simulink model "Dfig"  (R2014a)
settings: Solver=ode45  StartTime=0.0  StopTime=3.5  RelTol=1e-3
values from neighbouring files (symbols this model uses):
  Cbus = 80e-3    (= 0.08)    [Parameter_2M_DFIG.m]    (also in Parameter_2M_DFIG_GSC.m; ini2.m; init.m)
  D = 1e-3    (= 0.001)    [Parameter_2M_DFIG.m]    (also in Parameter_2M_DFIG_GSC.m = 0.1; ini.m; ini2.m; init.m)
  f = 50    [Parameter_2M_DFIG.m]    (also in Parameter_2M_DFIG_GSC.m = 60; ini.m; ini2.m; init.m)
  Fs = 1.28    [Parameter_2M_DFIG.m]    (also in Parameter_2M_DFIG_GSC.m = 1.8; ini.m = Vs*sqrt(2/3)/(2*pi*f); ini2.m = Vs*sqrt(2/3)/(2*pi*f); init.m = Vs*sqrt(2/3)/(2*pi*f))
  fsw = 4e3    (= 4000)    [Parameter_2M_DFIG.m]    (also in Parameter_2M_DFIG_GSC.m; ini.m; ini2.m; init.m)
  J = 127    [Parameter_2M_DFIG.m]    (also in Parameter_2M_DFIG_GSC.m = 90; ini.m; ini2.m; init.m)
  ki_id = (wni^2)*Lr*sigma    (= 491.599501999)    [Parameter_2M_DFIG.m]    (also in Parameter_2M_DFIG_GSC.m; ini.m; ini2.m; init.m)
  ki_idg = (wnig^2)*Lg    (= 68.6450725305)    [Parameter_2M_DFIG.m]    (also in Parameter_2M_DFIG_GSC.m; ini2.m = 56.8489213503; init.m = 56.8489213503)
  ki_iq = ki_id    (= 491.599501999)    [Parameter_2M_DFIG.m]    (also in Parameter_2M_DFIG_GSC.m; ini.m; ini2.m; init.m)
  ki_iqg = ki_idg    (= 68.6450725305)    [Parameter_2M_DFIG.m]    (also in Parameter_2M_DFIG_GSC.m; ini2.m = 56.8489213503; init.m = 56.8489213503)
  ki_n = ((wnn^2)*J)/p    (= 25400)    [Parameter_2M_DFIG.m]    (also in Parameter_2M_DFIG_GSC.m = 18000; ini.m; ini2.m; init.m)
  kp_id = (2*wni*sigma*Lr)-Rr    (= 0.5771)    [Parameter_2M_DFIG.m]    (also in Parameter_2M_DFIG_GSC.m; ini.m; ini2.m; init.m)
  kp_idg = (2*wnig*Lg)-Rg    (= 0.364153420404)    [Parameter_2M_DFIG.m]    (also in Parameter_2M_DFIG_GSC.m; ini2.m = 0.301572894745; init.m = 0.301572894745)
  kp_iq = kp_id    (= 0.5771)    [Parameter_2M_DFIG.m]    (also in Parameter_2M_DFIG_GSC.m; ini.m; ini2.m; init.m)
  kp_iqg = kp_idg    (= 0.364153420404)    [Parameter_2M_DFIG.m]    (also in Parameter_2M_DFIG_GSC.m; ini2.m = 0.301572894745; init.m = 0.301572894745)
  kp_n = (2*wnn*J)/p    (= 2540)    [Parameter_2M_DFIG.m]    (also in Parameter_2M_DFIG_GSC.m = 1800; ini.m; ini2.m; init.m)
  Kpg = 1/(1.5*Vs*sqrt(2/3))    [Parameter_2M_DFIG.m]    (also in Parameter_2M_DFIG_GSC.m; ini2.m; init.m)
  Kqg = -Kpg    [Parameter_2M_DFIG.m]    (also in Parameter_2M_DFIG_GSC.m; ini2.m; init.m)
  Lg = 483e-6    (= 0.000483)    [Parameter_2M_DFIG.m]    (also in Parameter_2M_DFIG_GSC.m; ini2.m = 0.0004; init.m = 0.0004)
  Lm = 2.5e-3    (= 0.0025)    [Parameter_2M_DFIG.m]    (also in Parameter_2M_DFIG_GSC.m; ini.m; ini2.m; init.m)
  Lr = Lm + Lsr    (= 0.002587)    [Parameter_2M_DFIG.m]    (also in Parameter_2M_DFIG_GSC.m; ini.m; ini2.m; init.m)
  Ls = Lm + Lsi    (= 0.002587)    [Parameter_2M_DFIG.m]    (also in Parameter_2M_DFIG_GSC.m; ini.m; ini2.m; init.m)
  Lsi = 87e-6    (= 8.7e-05)    [Parameter_2M_DFIG.m]    (also in Parameter_2M_DFIG_GSC.m; ini.m; ini2.m; init.m)
  N = 100    [Parameter_2M_DFIG.m]    (also in Parameter_2M_DFIG_GSC.m; ini2.m; init.m)
  p = 2    [Parameter_2M_DFIG.m]    (also in Parameter_2M_DFIG_GSC.m; ini.m; ini2.m; init.m)
  Ps = 2e6    (= 2000000)    [Parameter_2M_DFIG.m]    (also in Parameter_2M_DFIG_GSC.m; ini.m; ini2.m; init.m)
  Rg = 20e-6    (= 2e-05)    [Parameter_2M_DFIG.m]    (also in Parameter_2M_DFIG_GSC.m; ini2.m; init.m)
  Rr = 2.9e-3    (= 0.0029)    [Parameter_2M_DFIG.m]    (also in Parameter_2M_DFIG_GSC.m; ini.m; ini2.m; init.m)
  Rs = 2.6e-3    (= 0.0026)    [Parameter_2M_DFIG.m]    (also in Parameter_2M_DFIG_GSC.m; ini.m; ini2.m; init.m)
  sigma = 1- Lm^2/(Ls*Lr)    (= 0.0661284179513)    [Parameter_2M_DFIG.m]    (also in Parameter_2M_DFIG_GSC.m; ini.m; ini2.m; init.m)
  Tem = 12732    [Parameter_2M_DFIG.m]    (also in Parameter_2M_DFIG_GSC.m; ini.m; ini2.m; init.m)
  Ts = 1/fsw/f    (= 5e-06)    [Parameter_2M_DFIG.m]    (also in Parameter_2M_DFIG_GSC.m = 4.16666666667e-06; ini.m; ini2.m; init.m)
  Vbus = 1000    [Parameter_2M_DFIG.m]    (also in ini.m = Vr_stator*sqrt(2); ini2.m = 1150; init.m = 1150)
  Vs = 690    [Parameter_2M_DFIG.m]    (also in Parameter_2M_DFIG_GSC.m; ini.m; ini2.m; init.m)
undefined symbols (not defined in the file or in its folder): c1, c2, c3, c4, c5, c6, c7, c8, Ct, DiscIntNeverNeededParam, K1, K2
libraries: powerlib x18, powerlib_meascontrol x5, simulink x1
settings Model: CovSFcnEnable=on  Creator=admin  LastModifiedBy=admin
settings DebuggingCC: UnderspecifiedInitializationDetection=Classic  FrameProcessingCompatibilityMsg=error  StateNameClashWarn=warning
settings SimscapeCC: SimscapeNormalizeSystem=off
settings ConfigurationSet: Description=Simscape Multibody

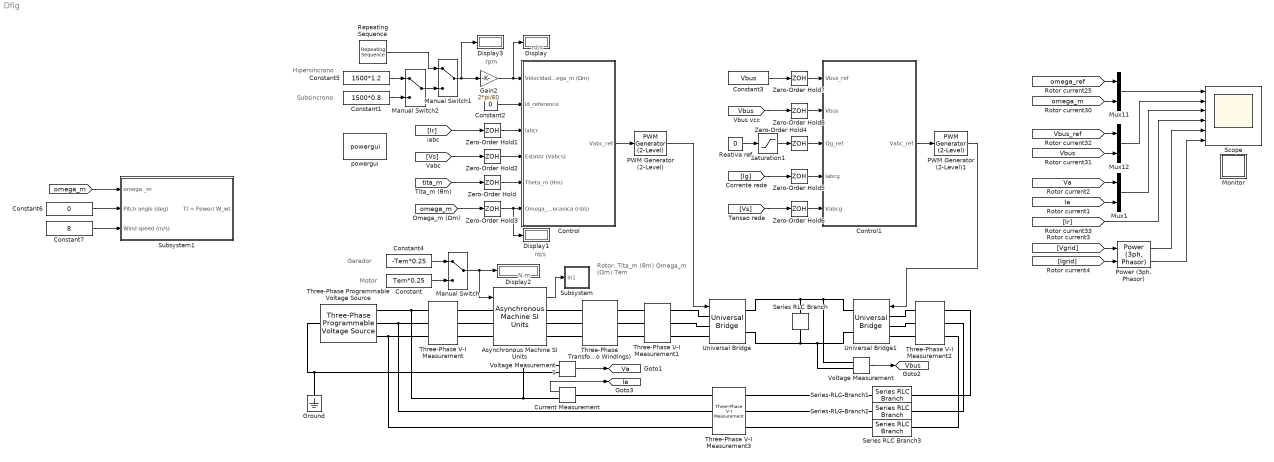
== system Dfig ==
  note: N.m
  note: Gerador
  note: Motor
  note: rd/s
  note: rpm
  note: Rotor:
      | Tita_m (θm)
      | Omega_m (Ωm)
      | Tem
  note: rd/s
  note: Hipersincrono
  note: Subsincrono
  Asynchronous Machine SI Units : powerlib/Machines/Asynchronous Machine SI Units  RotorType=Wound  PresetModel=No  MechanicalLoad=Torque Tm  ShowDetailedParameters=on  ReferenceFrame=Rotor  Units=SI  MeasurementBus=off  NominalParameters=[ Ps Vs f ]  Stator=[ Rs , Lsi]  Rotor=[ Rr , Lsi]  Cage1=[ 0.022 0.226/377]  Cage2=[ 0.022 0.226/377]  Lm=Lm  Mechanical=[ J D 2 ]  PolePairs=2  InitialConditions=[1 0 0 0 0 0 0 0]  SimulateSaturation=off  Saturation=[14.03593122, 27.81365428, 53.79336849, 72.68890987, 97.98006896, 148.6815601, 215.7428561, 302.9841135, 420.4778367 ; 230, 322, 414, 460, 506, 552, 598, 644, 690]  LoadFlowParameters=1492000  TsPowergui=0  TsBlock=-1  IterativeModel=Trapezoidal non iterative  IterativeDiscreteModel=Trapezoidal non iterative  Pmec=0
  Constant : Constant  Value=Tem*0.25
  Constant1 : Constant  Value=1500*0.8
  Constant2 : Constant  Value=0
  Constant3 : Constant  Value=Vbus
  Constant4 : Constant  Value=-Tem*0.25
  Constant5 : Constant  Value=1500*1.2
  Constant6 : Constant  Value=0
  Constant7 : Constant  Value=8
  Control : Subsystem
  Control1 : Subsystem
  Current Measurement : powerlib/Measurements/Current Measurement  PhasorSimulation=off  OutputType=Complex  PSBequivalent=0
  Display{,1..3} (4 alike) : Display
  Gain2 : Gain  Gain=2*pi/60
  Ground : powerlib/Elements/Ground  LConnTagsString=a
  Manual Switch : ManualSwitch
  Manual Switch1 : ManualSwitch
  Manual Switch2 : ManualSwitch
  Monitor : Subsystem
  Mux1 : Mux  Inputs=2
  Mux11 : Mux  Inputs=2
  Mux12 : Mux  Inputs=2
  PWM Generator (2-Level) : powerlib_meascontrol/Pulse & Signal Generators/PWM Generator (2-Level)  ModulatorType=Three-phase bridge (6 pulses)  ModulatorMode=Unsynchronized  Fc=fsw  Pc=0  nF=27  MinMax="[ -1  1 ]"  SamplingTechnique=Natural  ModulatingSignals=off  m=0.8  Freq=60  Phase=0  Ts=0  ShowCarrierOutport=off
  PWM Generator (2-Level)1 : powerlib_meascontrol/Pulse & Signal Generators/PWM Generator (2-Level)  ModulatorType=Three-phase bridge (6 pulses)  ModulatorMode=Unsynchronized  Fc=fsw  Pc=0  nF=27  MinMax="[ -1  1 ]"  SamplingTechnique=Natural  ModulatingSignals=off  m=0.8  Freq=60  Phase=0  Ts=0  ShowCarrierOutport=off
  "Power (3ph, Phasor)" : powerlib_meascontrol/Measurements/Power (3ph, Phasor)
  Reativa ref : Constant  Value=0
  Repeating Sequence : simulink/Sources/Repeating Sequence  rep_seq_t=[0 1.5 1.50001 2.5 2.50001 3.5]  rep_seq_y=1500*[0.8 0.8 1 1 1.2 1.2]
  Saturation1 : Saturate  UpperLimit=1000e3/2  LowerLimit=-1000e3/2
  Scope : Scope  NumInputPorts=6
      settings: TimeRange=auto  MaxDataPoints=5000  SaveToWorkspace=off  YMin=-24.02976~-364.64582~-7463.66317~-6632.25897~-2015970.8703~-1.00000  YMax=216.26787~3170.56911~4982.85673~5821.5871~2162882.51579~1.00000  SampleTime=-1
  Series RLC Branch : powerlib/Elements/Series RLC Branch  LConnTagsString=__new0  RConnTagsString=__new0  BranchType=C  Resistance=1  Inductance=1e-3  SetiL0=off  InitialCurrent=0  Capacitance=Cbus  Setx0=off  InitialVoltage=0  Measurements=Branch voltage
  Series RLC Branch1 : powerlib/Elements/Series RLC Branch  LConnTagsString=__new0  RConnTagsString=__new0  BranchType=RL  Resistance=Rg  Inductance=Lg  SetiL0=off  InitialCurrent=0  Capacitance=0  Setx0=off  InitialVoltage=0  Measurements=None
  Series RLC Branch2 : powerlib/Elements/Series RLC Branch  LConnTagsString=__new0  RConnTagsString=__new0  BranchType=RL  Resistance=Rg  Inductance=Lg  SetiL0=off  InitialCurrent=0  Capacitance=0  Setx0=off  InitialVoltage=0  Measurements=None
  Series RLC Branch3 : powerlib/Elements/Series RLC Branch  LConnTagsString=__new0  RConnTagsString=__new0  BranchType=RL  Resistance=Rg  Inductance=Lg  SetiL0=off  InitialCurrent=0  Capacitance=0  Setx0=off  InitialVoltage=0  Measurements=None
  Subsystem : Subsystem
  Subsystem1 : Subsystem
  Three-Phase Programmable Voltage Source : powerlib/Electrical Sources/Three-Phase Programmable Voltage Source  PositiveSequence="[Vs  0 f]"  VariationEntity=None  VariationType=Table of time-amplitude pairs  VariationTypeAlt=Step  VariationStep=0.5  VariationRate=10  VariationMagnitude=0.3  VariationFrequency=2  VariationTiming=[1 2]  VariationPhaseA=off  Amplitudes=[1 0.8 1.2 1.0]  TimeValues=[0 0.1 0.15 0.2]  HarmonicGeneration=off  HarmonicA=[3 0.2 -25 0]  HarmonicB=[2 0.15 35 2]  Timing="[0.05  3]"  BusType=swing  Pref=0  Qref=0  Qmin=-inf  Qmax=inf
  Three-Phase Transformer (Two Windings) : powerlib/Elements/Three-Phase Transformer (Two Windings)  Winding1Connection=Y  Winding2Connection=Y  CoreType=Three single-phase transformers  SetSaturation=off  Hysteresis=off  DataFile='hysteresis'  SetInitialFlux=off  Measurements=None  UNITS=SI  NominalPower=[ Ps , f]  Winding1=[Vs 0 0]  Winding2=[Vs/u 0 0]  Rm=1.0805e+06  Lm=2866  L0=0.5  Saturation=[0 0;0.66653 1910.3;277.72 2419.7]  InitialFluxes=[1273.5 -1273.5 1114.3]  MoreParameters=off  BreakLoop=off  DataType=on  TransfoNumber=1
  Three-Phase V-I Measurement : powerlib/Measurements/Three-Phase V-I Measurement  VoltageMeasurement=phase-to-ground  SetLabelV=on  LabelV=Vs  Vpu=off  VpuLL=off  CurrentMeasurement=yes  SetLabelI=on  LabelI=Is  Ipu=off  Pbase=100e6  Vbase=500e3  OutputType=Complex  PhasorSimulation=off  PSBequivalent=0
  Three-Phase V-I Measurement1 : powerlib/Measurements/Three-Phase V-I Measurement  VoltageMeasurement=phase-to-phase  SetLabelV=on  LabelV=Vr  Vpu=off  VpuLL=off  CurrentMeasurement=yes  SetLabelI=on  LabelI=Ir  Ipu=off  Pbase=100e6  Vbase=500e3  OutputType=Complex  PhasorSimulation=off  PSBequivalent=0
  Three-Phase V-I Measurement2 : powerlib/Measurements/Three-Phase V-I Measurement  VoltageMeasurement=no  SetLabelV=on  LabelV=Vg  Vpu=off  VpuLL=off  CurrentMeasurement=yes  SetLabelI=on  LabelI=Ig  Ipu=off  Pbase=100e6  Vbase=500e3  OutputType=Complex  PhasorSimulation=off  PSBequivalent=0
  Three-Phase V-I Measurement3 : powerlib/Measurements/Three-Phase V-I Measurement  VoltageMeasurement=phase-to-phase  SetLabelV=on  LabelV=Vgrid  Vpu=off  VpuLL=off  CurrentMeasurement=yes  SetLabelI=on  LabelI=Igrid  Ipu=off  Pbase=100e6  Vbase=500e3  OutputType=Complex  PhasorSimulation=off  PSBequivalent=0
  Universal Bridge : powerlib/Power Electronics/Universal Bridge  Arms=3  SnubberResistance=1e5  SnubberCapacitance=inf  Device=Ideal Switches  Ron=1e-3  Lon=0  ForwardVoltages="[  0  0  ]"  ForwardVoltage=0  GTOparameters=[ 10e-6 , 20e-6 ]  IGBTparameters=[ 1e-6 , 2e-6 ]  Measurements=None  Measurements_2=None  converterType=Rectifier
  Universal Bridge1 : powerlib/Power Electronics/Universal Bridge  Arms=3  SnubberResistance=1e5  SnubberCapacitance=inf  Device=Ideal Switches  Ron=1e-3  Lon=0  ForwardVoltages="[  0  0  ]"  ForwardVoltage=0  GTOparameters=[ 10e-6 , 20e-6 ]  IGBTparameters=[ 1e-6 , 2e-6 ]  Measurements=None  Measurements_2=None  converterType=Rectifier
  Voltage Measurement : powerlib/Measurements/Voltage Measurement  PhasorSimulation=off  OutputType=Complex  PSBequivalent=0
  Voltage Measurement1 : powerlib/Measurements/Voltage Measurement  PhasorSimulation=off  OutputType=Complex  PSBequivalent=0
  Zero-Order Hold{,1..8} (9 alike) : ZeroOrderHold  SampleTime=1/fsw
  powergui : powerlib/powergui  Priority=1  SimulationMode=Discrete  SampleTime=Ts  frequency=60  Iterations=50  frequencyindice=50  Pbase=100e6  ErrMax=1e-4  UnitsV=kV  UnitsW=MW  buscounter=0  FunctionMessages=off  echomessages=off  EnableUseOfTLC=off  CurrentSourceSwitches=off  DisableSnubberDevices=off  DisableRonSwitches=off  DisableVfSwitches=off  DisplayEquations=off  SolverType=Tustin  Interpol=off  ExternalGateDelay=off  methode=off  Ts=0  x0status=blocks  SPID=off  SwTol=0  HookPort=off  RestoreLinks=warning  ResistiveCurrentMeasurement=off  Frange=[0:2:500]  Ylog=off  Xlog=on  ShowGrid=off  save=off  variable=ZData  structure=0  ZoomFFT=off  StartTime=0.0  cycles=1  DisplayStyle=1  fundamental=60  FreqAxis=off  MaxFrequency=1000  frequencyindicesteady=1  RmsSteady=1  display=off
  tag scope: Ia=global, Va=global, Vbus=global
  wires:
  PWM Generator (2-Level)/1 -> Universal Bridge/1
  Control/1(Vabc_ref) -> PWM Generator (2-Level)/1
  Constant2/1 -> Control/2(id_reference)
  [Vs] -> Zero-Order Hold2/1
  [Ir] -> Zero-Order Hold1/1
  Asynchronous Machine SI Units/1 -> Subsystem/1(In1)
  [tita_m] -> Zero-Order Hold/1
  [omega_m] -> Zero-Order Hold3/1
  Zero-Order Hold1/1 -> Control/3(iabcr)
  Zero-Order Hold2/1 -> Control/4(Estator (Vabcs))
  Zero-Order Hold/1 -> Control/5(Theta_m (θm))
  Zero-Order Hold3/1 -> Display1/1, Control/6(Omega_m (Ωm) Mecanica (rd/s))
  Gain2/1 -> Display/1, Control/1("Velocidade ref (rd/s) Omega_m (Ωm) ")
  [Ig] -> Zero-Order Hold5/1
  [Vs] -> Zero-Order Hold6/1
  Constant3/1 -> Zero-Order Hold7/1
  Zero-Order Hold6/1 -> Control1/5("Vabcg ")
  Zero-Order Hold5/1 -> Control1/4(iabcg)
  Reativa ref/1 -> Saturation1/1
  Zero-Order Hold4/1 -> Control1/3(Qg_ref)
  Zero-Order Hold7/1 -> Control1/1(Vbus_ref)
  Saturation1/1 -> Zero-Order Hold4/1
  [Vbus] -> Zero-Order Hold8/1
  Zero-Order Hold8/1 -> Control1/2(Vbus)
  Control1/1(Vabc_ref) -> PWM Generator (2-Level)1/1
  PWM Generator (2-Level)1/1 -> Universal Bridge1/1
  Voltage Measurement/1 -> [Vbus]
  Voltage Measurement1/1 -> [Va]
  [omega_m] -> Mux11/2
  [Vbus_ref] -> Mux12/1
  [Vbus] -> Mux12/2
  [omega_ref] -> Mux11/1
  [Ia] -> Mux1/2
  [Va] -> Mux1/1
  Mux11/1 -> Scope/1
  Mux12/1 -> Scope/2
  Mux1/1 -> Scope/3
  [Ir] -> Scope/4
  Constant/1 -> Manual Switch/2
  Constant4/1 -> Manual Switch/1
  Manual Switch/1 -> Display2/1, Asynchronous Machine SI Units/1
  Manual Switch1/1 -> Display3/1, Gain2/1
  Constant5/1 -> Manual Switch2/1
  Constant1/1 -> Manual Switch2/2
  Manual Switch2/1 -> Manual Switch1/2
  Current Measurement/1 -> [Ia]
  [Igrid] -> "Power (3ph, Phasor)"/2
  [Vgrid] -> "Power (3ph, Phasor)"/1
  "Power (3ph, Phasor)"/1 -> Scope/5
  "Power (3ph, Phasor)"/2 -> Scope/6
  Repeating Sequence/1 -> Manual Switch1/1
  [omega_m] -> Subsystem1/1(omega _m)
  Constant7/1 -> Subsystem1/3(Wind speed (m/s))
  Constant6/1 -> Subsystem1/2(Pitch angle (deg))
  connections:
  Three-Phase Programmable Voltage Source/LConn1 -- Voltage Measurement1/LConn2 -- Ground/LConn1
  Voltage Measurement1/LConn1 -- Current Measurement/RConn1 -- Three-Phase Programmable Voltage Source/RConn1 -- Three-Phase V-I Measurement/LConn1
  Three-Phase Programmable Voltage Source/RConn3 -- Three-Phase V-I Measurement3/RConn3 -- Three-Phase V-I Measurement/LConn3
  Asynchronous Machine SI Units/LConn1 -- Three-Phase V-I Measurement/RConn1
  Asynchronous Machine SI Units/LConn2 -- Three-Phase V-I Measurement/RConn2
  Asynchronous Machine SI Units/LConn3 -- Three-Phase V-I Measurement/RConn3
  Three-Phase V-I Measurement1/LConn1 -- Universal Bridge/LConn1
  Three-Phase V-I Measurement1/LConn2 -- Universal Bridge/LConn2
  Three-Phase V-I Measurement1/LConn3 -- Universal Bridge/LConn3
  Universal Bridge/RConn1 -- Series RLC Branch/LConn1 -- Voltage Measurement/LConn1 -- Universal Bridge1/RConn1
  Universal Bridge/RConn2 -- Series RLC Branch/RConn1 -- Voltage Measurement/LConn2 -- Universal Bridge1/RConn2
  Universal Bridge1/LConn1 -- Three-Phase V-I Measurement2/LConn1
  Universal Bridge1/LConn2 -- Three-Phase V-I Measurement2/LConn2
  Universal Bridge1/LConn3 -- Three-Phase V-I Measurement2/LConn3
  Three-Phase V-I Measurement2/RConn1 -- Series RLC Branch1/LConn1
  Three-Phase V-I Measurement2/RConn2 -- Series RLC Branch2/LConn1
  Three-Phase V-I Measurement2/RConn3 -- Series RLC Branch3/LConn1
  Asynchronous Machine SI Units/RConn2 -- Three-Phase Transformer (Two Windings)/LConn2
  Asynchronous Machine SI Units/RConn3 -- Three-Phase Transformer (Two Windings)/LConn3
  Three-Phase Transformer (Two Windings)/RConn1 -- Three-Phase V-I Measurement1/RConn1
  Three-Phase Transformer (Two Windings)/RConn2 -- Three-Phase V-I Measurement1/RConn2
  Three-Phase Transformer (Two Windings)/RConn3 -- Three-Phase V-I Measurement1/RConn3
  Three-Phase Transformer (Two Windings)/LConn1 -- Asynchronous Machine SI Units/RConn1
  Three-Phase Programmable Voltage Source/RConn2 -- Three-Phase V-I Measurement3/RConn2 -- Three-Phase V-I Measurement/LConn2
  Three-Phase V-I Measurement3/LConn1 -- Series RLC Branch1/RConn1
  Three-Phase V-I Measurement3/LConn2 -- Series RLC Branch2/RConn1
  Three-Phase V-I Measurement3/LConn3 -- Series RLC Branch3/RConn1
  Three-Phase V-I Measurement3/RConn1 -- Current Measurement/LConn1

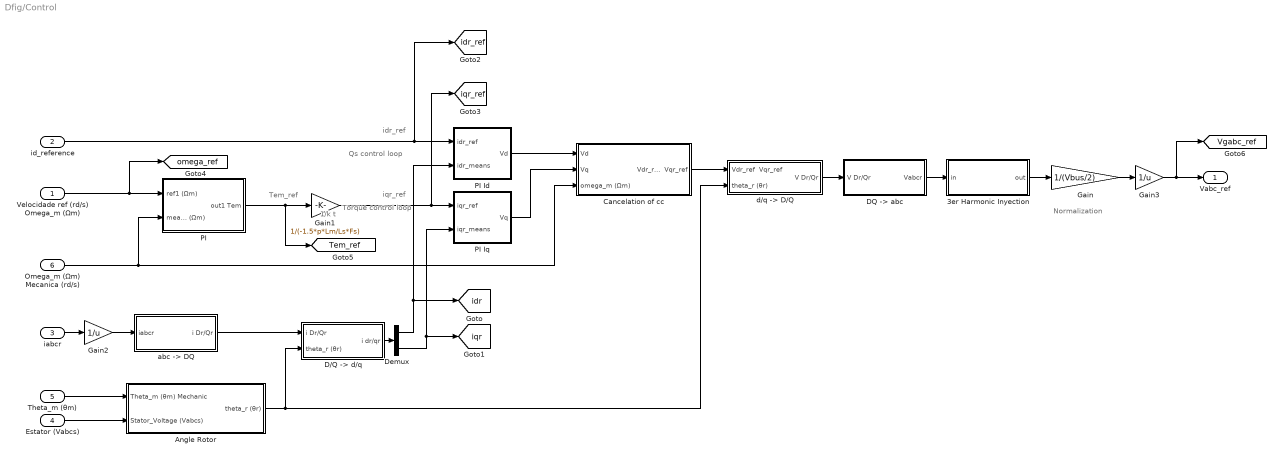
== system Dfig/Control ==
  note: Normalization
  note: Torque control loop
  note: 1/k t
  note: iqr_ref
  note: Tem_ref
  note: idr_ref
  note: Qs control loop
  "Velocidade ref (rd/s) Omega_m (Ωm) " : Inport
  id_reference : Inport  Port=2
  iabcr : Inport  Port=3
  Estator (Vabcs) : Inport  Port=4
  Theta_m (θm) : Inport  Port=5
  Omega_m (Ωm) Mecanica (rd/s) : Inport  Port=6
  " Angle Rotor" : Subsystem
  3er Harmonic Inyection : Subsystem
  Cancelation of cc : Subsystem
  "D/Q -> d/q" : Subsystem
  "DQ -> abc" : Subsystem
  Demux : Demux  Outputs=2
  Gain : Gain  Gain=1/(Vbus/2)
  Gain1 : Gain  Gain=1/(-1.5*p*Lm/Ls*Fs)
  Gain2 : Gain  Gain=1/u
  Gain3 : Gain  Gain=1/u
  PI : Subsystem
  PI Id : Subsystem
  PI Iq : Subsystem
  "abc -> DQ " : Subsystem
  "d/q -> D/Q " : Subsystem
  Vabc_ref : Outport
  tag scope: Tem_ref=global, Vgabc_ref=global, idr=global, idr_ref=global, iqr=global, iqr_ref=global, omega_ref=global
  wires:
  "DQ -> abc"/1(Vabcr) -> 3er Harmonic Inyection/1(in)
  "d/q -> D/Q "/1(V Dr/Qr) -> "DQ -> abc"/1(V Dr/Qr)
  iabcr/1 -> Gain2/1
  "abc -> DQ "/1(i Dr/Qr) -> "D/Q -> d/q"/1(i Dr/Qr)
  3er Harmonic Inyection/1(out) -> Gain/1
  Theta_m (θm)/1 -> " Angle Rotor"/1(Theta_m (θm) Mechanic)
  Estator (Vabcs)/1 -> " Angle Rotor"/2(Stator_Voltage (Vabcs))
  " Angle Rotor"/1(theta_r (θr)) -> "D/Q -> d/q"/2(theta_r (θr)), "d/q -> D/Q "/2(theta_r (θr))
  PI Id/1(Vd) -> Cancelation of cc/1(Vd)
  PI Iq/1(Vq) -> Cancelation of cc/2(Vq)
  Omega_m (Ωm) Mecanica (rd/s)/1 -> PI/2("means1 (Ωm) "), Cancelation of cc/3(omega_m (Ωm))
  "D/Q -> d/q"/1(i dr/qr) -> Demux/1
  Demux/2 -> [iqr], PI Iq/2(iqr_means)
  Demux/1 -> [idr], PI Id/2(idr_means)
  PI/1(out1 Tem) -> [Tem_ref], Gain1/1
  Gain1/1 -> [iqr_ref], PI Iq/1(iqr_ref)
  id_reference/1 -> [idr_ref], PI Id/1(idr_ref)
  Cancelation of cc/1(Vdr_ref  Vqr_ref) -> "d/q -> D/Q "/1(Vdr_ref  Vqr_ref)
  "Velocidade ref (rd/s) Omega_m (Ωm) "/1 -> [omega_ref], PI/1("ref1 (Ωm) ")
  Gain/1 -> Gain3/1
  Gain2/1 -> "abc -> DQ "/1(iabcr)
  Gain3/1 -> [Vgabc_ref], Vabc_ref/1

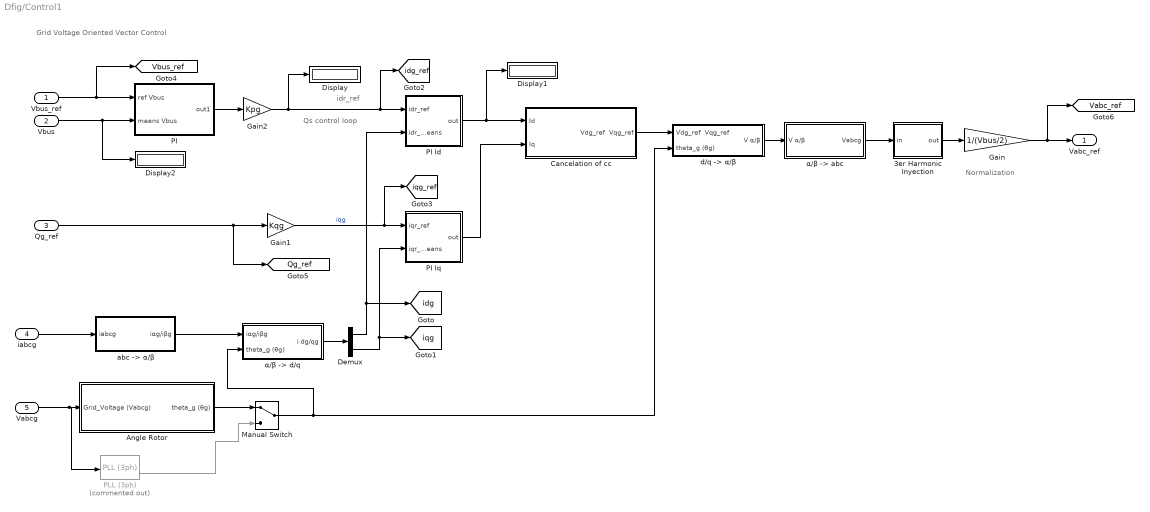
== system Dfig/Control1 ==
  note: Qs control loop
  note: idr_ref
  note: Normalization
  note: Grid Voltage Oriented Vector Control
  Vbus_ref : Inport
  Vbus : Inport  Port=2
  Qg_ref : Inport  Port=3
  iabcg : Inport  Port=4
  "Vabcg " : Inport  Port=5
  " Angle Rotor" : Subsystem
  3er Harmonic Inyection : Subsystem
  Cancelation of cc : Subsystem
  Demux : Demux  Outputs=2
  Display : Display
  Display1 : Display
  Display2 : Display
  Gain : Gain  Gain=1/(Vbus/2)
  Gain1 : Gain  Gain=Kqg
  Gain2 : Gain  Gain=Kpg
  Manual Switch : ManualSwitch
  PI : Subsystem
  PI Id : Subsystem
  PI Iq : Subsystem
  PLL (3ph) : powerlib_meascontrol/PLL/PLL (3ph)  Commented=on  Fmin=45  Par_Init=[0, 60]  ParK=[180, 3200, 1]  TcD=1e-4  MaxRateChangeFreq=12  FilterCutOffFreq=25  Ts=0  AGC=on
      link override Model/abc to dq0: Alignment=Aligned with phase A axis
  "abc -> α/β " : Subsystem
  "d/q -> α/β " : Subsystem
  "α/β -> abc" : Subsystem
  "α/β -> d/q" : Subsystem
  Vabc_ref : Outport
  tag scope: Qg_ref=global, Vabc_ref=global, Vbus_ref=global, idg=global, idg_ref=global, iqg=global, iqg_ref=global
  wires:
  Gain/1 -> Vabc_ref/1, [Vabc_ref]
  Cancelation of cc/1(Vdg_ref  Vqg_ref) -> "d/q -> α/β "/1(Vdg_ref  Vqg_ref)
  Gain1/1 -> PI Iq/1(iqr_ref), [iqg_ref]  "iqg"
  Demux/1 -> PI Id/2(idr_means), [idg]
  Demux/2 -> PI Iq/2(iqr_means), [iqg]
  PI Iq/1(out) -> Cancelation of cc/2(Iq)
  PI Id/1(out) -> Display1/1, Cancelation of cc/1(Id)
  3er Harmonic Inyection/1(out) -> Gain/1
  "abc -> α/β "/1(iαg/iβg) -> "α/β -> d/q"/1(iαg/iβg)
  "d/q -> α/β "/1(V α/β) -> "α/β -> abc"/1(V α/β)
  iabcg/1 -> "abc -> α/β "/1(iabcg)
  Vbus_ref/1 -> [Vbus_ref], PI/1("ref Vbus ")
  Gain2/1 -> Display/1, [idg_ref], PI Id/1(idr_ref)
  Vbus/1 -> Display2/1, PI/2("means Vbus ")
  Qg_ref/1 -> [Qg_ref], Gain1/1
  "α/β -> abc"/1(Vabcg) -> 3er Harmonic Inyection/1(in)
  "Vabcg "/1 -> PLL (3ph)/1, " Angle Rotor"/1(Grid_Voltage (Vabcg))
  PI/1(out1) -> Gain2/1
  " Angle Rotor"/1(theta_g (θg)) -> Manual Switch/1
  Manual Switch/1 -> "α/β -> d/q"/2(theta_g (θg)), "d/q -> α/β "/2(theta_g (θg))
  "α/β -> d/q"/1(i dg/qg) -> Demux/1
  PLL (3ph)/2 -> Manual Switch/2

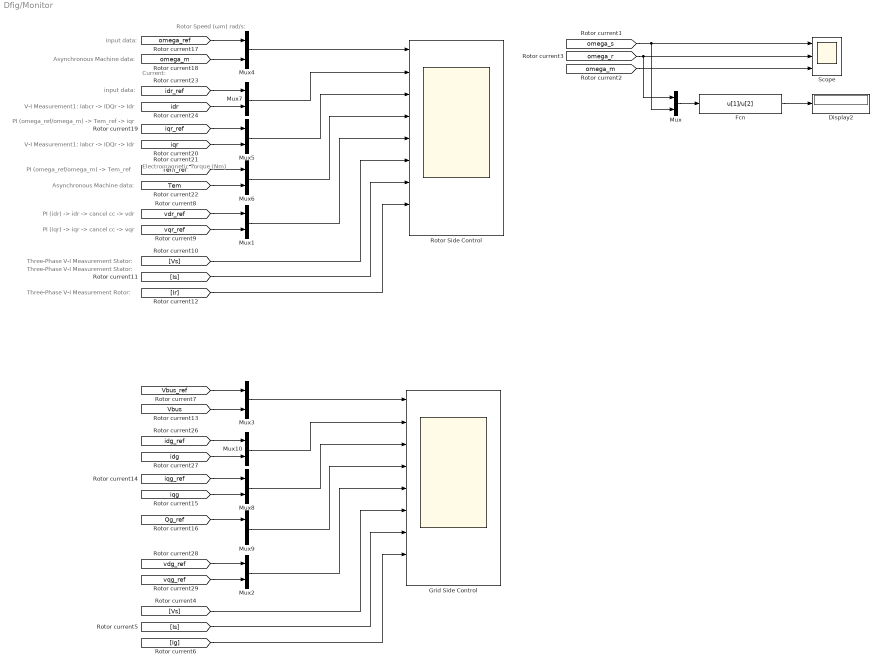
== system Dfig/Monitor ==
  note: Electromagnetic Torque (Nm)
  note: Three-Phase V-I Measurement Stator:
  note: PI (idr) -> idr -> cancel cc -> vdr
  note: PI (omega_ref/omega_m) -> Tem_ref -> iqr
  note: V-I Measurement1: Iabcr -> IDQr -> Idr
  note: input data:
  note: Current:
  note: Rotor Speed (ωm) rad/s:
  note: Asynchronous Machine data:
  note: input data:
  note: V-I Measurement1: Iabcr -> IDQr -> Idr
  note: PI (omega_ref/omega_m) -> Tem_ref
  note: Asynchronous Machine data:
  note: PI (iqr) -> iqr -> cancel cc -> vqr
  note: Three-Phase V-I Measurement Stator:
  note: Three-Phase V-I Measurement Rotor:
  Display2 : Display
  Fcn : Fcn  Expr=u[1]/u[2]
  Grid Side Control : Scope  NumInputPorts=9
      settings: TimeRange=auto  MaxDataPoints=5000  SaveToWorkspace=off  SaveName=ScopeData2  YMin=-364.63596~-4571.81946~-2149.77113~-1.00000~-1423.80446~-704.2283~-17831.01804~-7699.57837~-1.00000  YMax=3170.48037~3435.16431~6550.53156~1.00000~1318.4789~704.2283~20396.17506~7110.81698~1.00000  SampleInput=on  SampleTime=5e-5
  Mux{,1..10} (11 alike) : Mux  Inputs=2
  Rotor Side Control : Scope  NumInputPorts=9
      settings: TimeRange=auto  MaxDataPoints=5000  SaveToWorkspace=off  SaveName=ScopeData3  YMin=-24.06947~-3472.34631~-13143.18045~-28029.84842~-1231.01694~-704.2283~-17831.01804~-6632.23462~-1.00000  YMax=216.62525~1402.42703~5272.58533~86610.1332~1394.74885~704.2283~20396.17506~5821.53238~1.00000  SampleInput=on  SampleTime=5e-5
  Scope : Scope  NumInputPorts=3
      settings: TimeRange=auto  MaxDataPoints=5000  SaveToWorkspace=off  YMin=-118.37647~-5~-5  YMax=362.21879~5~5  SampleTime=-1
  wires:
  [omega_m] -> Mux4/2
  [omega_ref] -> Mux4/1
  [iqr_ref] -> Mux5/1
  [iqr] -> Mux5/2
  [Tem_ref] -> Mux6/1
  [idr] -> Mux7/2
  [idr_ref] -> Mux7/1
  Mux4/1 -> Rotor Side Control/1
  [vdr_ref] -> Mux1/1
  [vqr_ref] -> Mux1/2
  Mux7/1 -> Rotor Side Control/2
  Mux5/1 -> Rotor Side Control/3
  Mux6/1 -> Rotor Side Control/4
  Mux1/1 -> Rotor Side Control/5
  [Vs] -> Rotor Side Control/6
  [Is] -> Rotor Side Control/7
  [Ir] -> Rotor Side Control/8
  [Tem] -> Mux6/2
  [omega_m] -> Scope/3
  [omega_r] -> Mux/1, Scope/2
  Fcn/1 -> Display2/1
  Mux/1 -> Fcn/1
  [omega_s] -> Mux/2, Scope/1
  [Ig] -> Grid Side Control/8
  [Is] -> Grid Side Control/7
  [Vs] -> Grid Side Control/6
  Mux2/1 -> Grid Side Control/5
  Mux9/1 -> Grid Side Control/4
  Mux8/1 -> Grid Side Control/3
  Mux10/1 -> Grid Side Control/2
  [vqg_ref] -> Mux2/2
  [vdg_ref] -> Mux2/1
  Mux3/1 -> Grid Side Control/1
  [idg_ref] -> Mux10/1
  [idg] -> Mux10/2
  [Qg_ref] -> Mux9/1
  [iqg] -> Mux8/2
  [iqg_ref] -> Mux8/1
  [Vbus_ref] -> Mux3/1
  [Vbus] -> Mux3/2

== system Dfig/Subsystem ==
  In1 : Inport
  Bus Selector : BusSelector  OutputSignals=Mechanical.Rotor angle thetam (rad),Mechanical.Rotor speed (wm),Mechanical.Electromagnetic torque Te (N*m)
  tag scope: Tem=global, omega_m=global, tita_m=global
  wires:
  Bus Selector/2 -> [omega_m]  "<Rotor speed (wm)>"
  In1/1 -> Bus Selector/1
  Bus Selector/1 -> [tita_m]  "<Rotor angle thetam (rad)>"
  Bus Selector/3 -> [Tem]  "<Electromagnetic torque Te (N*m)>"

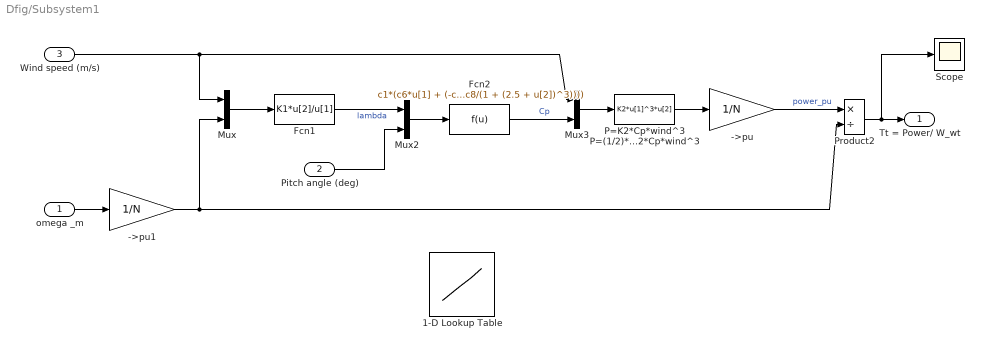
== system Dfig/Subsystem1 ==
  omega _m : Inport
  Pitch angle (deg) : Inport  Port=2
  Wind speed (m/s) : Inport  Port=3
  ->pu : Gain  Gain=1/N
  ->pu1 : Gain  Gain=1/N
  1-D Lookup Table : Lookup_n-D  NumberOfTableDimensions=1  BreakpointsForDimension1=[01:0.01:11.8]  Table=Ct  InternalRulePriority=Speed  RndMeth=Simplest  InputSameDT=on
  Fcn1 : Fcn  Expr=K1*u[2]/u[1]
  Fcn2 : Fcn  Expr=c1*(c6*u[1] + (-c4 - c3*(2.5 + u[2]) + c2*(1/(u[1] + c7*(2.5 + u[2])) -c8/(1 + (2.5 + u[2])^3)))/exp(c5*(1/(u[1] + c7*(2.5 + u[2])) - c8/(1 + (2.5 + u[2])^3))))
  Mux : Mux  Inputs=2
  Mux2 : Mux  Inputs=2
  Mux3 : Mux  Inputs=2
  P=K2*Cp*wind^3 P=(1/2)*pi*densidad*radio^2*Cp*wind^3 : Fcn  Expr=K2*u[1]^3*u[2]
  Product2 : Product  Inputs=*/  SaturateOnIntegerOverflow=on  InputSameDT=on  OutDataTypeStr=Inherit: Same as first input
  Scope : Scope
      settings: TimeRange=auto  MaxDataPoints=5000  SaveToWorkspace=off  YMin=-10  YMax=10  SampleTime=-1
  Tt = Power/ W_wt : Outport
  wires:
  Wind speed (m/s)/1 -> Mux/1, Mux3/1
  Product2/1 -> Scope/1, Tt = Power/ W_wt/1
  Mux3/1 -> P=K2*Cp*wind^3 P=(1/2)*pi*densidad*radio^2*Cp*wind^3/1
  Fcn2/1 -> Mux3/2  "Cp"
  Pitch angle (deg)/1 -> Mux2/2
  ->pu/1 -> Product2/1  "power_pu"
  Fcn1/1 -> Mux2/1  "lambda"
  omega _m/1 -> ->pu1/1
  Mux/1 -> Fcn1/1
  P=K2*Cp*wind^3 P=(1/2)*pi*densidad*radio^2*Cp*wind^3/1 -> ->pu/1
  Mux2/1 -> Fcn2/1
  ->pu1/1 -> Mux/2, Product2/2

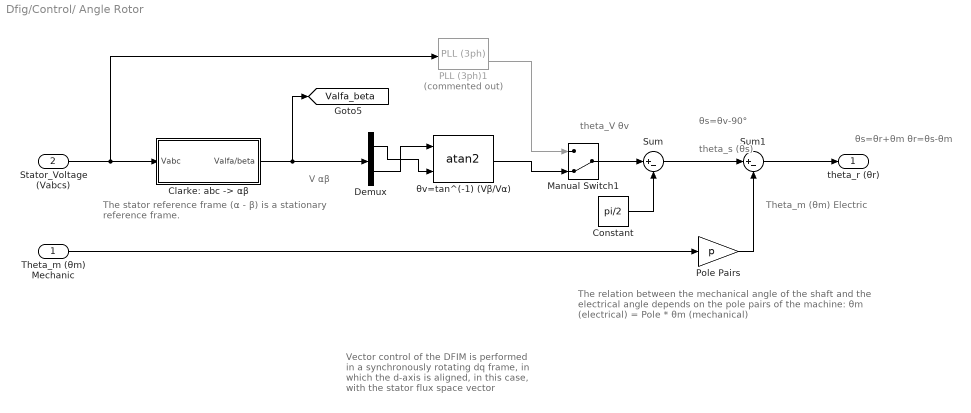
== system Dfig/Control/ Angle Rotor ==
  note: Theta_m (θm)
      | Electric
  note: theta_V θv
  note: The stator reference frame (α - β) is a stationary
      | reference frame.
  note: The relation between the mechanical angle of the shaft and the
      | electrical angle depends on the pole pairs of the machine:
      |
      | θm (electrical) = Pole * θm (mechanical)
  note: theta_s (θs)
  note: V αβ
  note: θs=θv-90°
  note: θs=θr+θm
      | θr=θs-θm
  note: Vector control of the DFIM is performed in a synchronously rotating dq frame, in which the d-axis is aligned, in this case, with the stator flux space vector
  Theta_m (θm) Mechanic : Inport
  Stator_Voltage (Vabcs) : Inport  Port=2
  "Clarke: abc -> αβ " : Subsystem
  Constant : Constant  Value=pi/2
  Demux : Demux  Outputs=2
  Manual Switch1 : ManualSwitch  CurrentSetting=0
  PLL (3ph)1 : powerlib_meascontrol/PLL/PLL (3ph)  Commented=on  Fmin=45  Par_Init=[0, 60]  ParK=[180, 3200, 1]  TcD=1e-4  MaxRateChangeFreq=12  FilterCutOffFreq=25  Ts=0  AGC=on
      link override Model/abc to dq0: Alignment=Aligned with phase A axis
  Pole Pairs : Gain  Gain=p
  Sum : Sum  Inputs=|+-
  Sum1 : Sum  Inputs=|+-
  θv=tan^(-1) (Vβ/Vα) : Trigonometry  Operator=atan2
  theta_r (θr) : Outport
  tag scope: Valfa_beta=global
  wires:
  Stator_Voltage (Vabcs)/1 -> PLL (3ph)1/1, "Clarke: abc -> αβ "/1(Vabc)
  Demux/2 -> θv=tan^(-1) (Vβ/Vα)/1
  Demux/1 -> θv=tan^(-1) (Vβ/Vα)/2
  "Clarke: abc -> αβ "/1("Valfa/beta ") -> Demux/1, [Valfa_beta]
  Constant/1 -> Sum/2
  Theta_m (θm) Mechanic/1 -> Pole Pairs/1
  Sum/1 -> Sum1/1
  Sum1/1 -> theta_r (θr)/1
  Pole Pairs/1 -> Sum1/2
  Manual Switch1/1 -> Sum/1
  θv=tan^(-1) (Vβ/Vα)/1 -> Manual Switch1/2
  PLL (3ph)1/2 -> Manual Switch1/1

== system Dfig/Control/3er Harmonic Inyection ==
  in : Inport
  Gain : Gain  Gain=-0.5
  MinMax : MinMax
  MinMax1 : MinMax  Function=max
  Scope : Scope
      settings: TimeRange=auto  MaxDataPoints=5000  SaveToWorkspace=off  SaveName=ScopeData2  YMin=-208.5095  YMax=235.47421  SampleTime=-1
  Sum : Sum  Inputs=|++
  Sum1 : Sum  Inputs=|++
  out : Outport
  wires:
  in/1 -> Sum1/1, MinMax1/1, MinMax/1
  MinMax/1 -> Sum/1
  MinMax1/1 -> Sum/2
  Sum1/1 -> out/1
  Sum/1 -> Gain/1
  Gain/1 -> Scope/1, Sum1/2

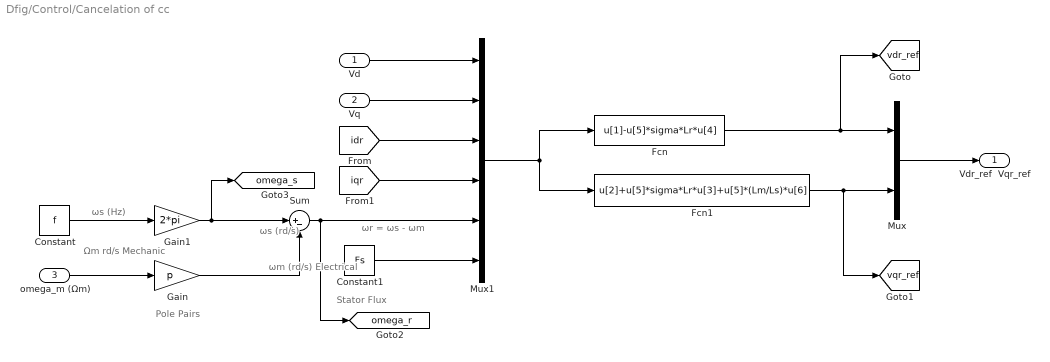
== system Dfig/Control/Cancelation of cc ==
  note: Stator Flux
  note: Ωm rd/s
      | Mechanic
  note: ωs (Hz)
  note: Pole Pairs
  note: ωr = ωs - ωm
  note: ωs (rd/s)
  note: ωm (rd/s)
      | Electrical
  Vd : Inport
  Vq : Inport  Port=2
  omega_m (Ωm) : Inport  Port=3
  Constant : Constant  Value=f
  Constant1 : Constant  Value=Fs
  Fcn : Fcn  Expr=u[1]-u[5]*sigma*Lr*u[4]
  Fcn1 : Fcn  Expr=u[2]+u[5]*sigma*Lr*u[3]+u[5]*(Lm/Ls)*u[6]
  Gain : Gain  Gain=p
  Gain1 : Gain  Gain=2*pi
  Mux : Mux  Inputs=2
  Mux1 : Mux  Inputs=6
  Sum : Sum  Inputs=|+-
  Vdr_ref  Vqr_ref : Outport
  tag scope: omega_r=global, omega_s=global, vdr_ref=global, vqr_ref=global
  wires:
  Mux/1 -> Vdr_ref  Vqr_ref/1
  Fcn/1 -> [vdr_ref], Mux/1
  Fcn1/1 -> [vqr_ref], Mux/2
  Vd/1 -> Mux1/1
  Vq/1 -> Mux1/2
  Mux1/1 -> Fcn1/1, Fcn/1
  [idr] -> Mux1/3
  [iqr] -> Mux1/4
  Constant1/1 -> Mux1/6
  omega_m (Ωm)/1 -> Gain/1
  Gain/1 -> Sum/2
  Constant/1 -> Gain1/1
  Gain1/1 -> [omega_s], Sum/1
  Sum/1 -> [omega_r], Mux1/5

== system Dfig/Control/D//Q -> d//q ==
  i Dr/Qr : Inport
  theta_r (θr) : Inport  Port=2
  Fcn : Fcn  Expr=u(1)*cos(u[3])+u[2]*sin(u[3])
  Fcn1 : Fcn  Expr=-u(1)*sin(u[3])+u[2]*cos(u[3])
  Mux : Mux  Inputs=2
  Mux1 : Mux  Inputs=2
  i dr/qr : Outport
  wires:
  Mux/1 -> i dr/qr/1
  Fcn/1 -> Mux/1
  Fcn1/1 -> Mux/2
  i Dr/Qr/1 -> Mux1/1
  theta_r (θr)/1 -> Mux1/2
  Mux1/1 -> Fcn1/1, Fcn/1

== system Dfig/Control/DQ -> abc ==
  V Dr/Qr : Inport
  Fcn : Fcn  Expr=u(1)
  Fcn1 : Fcn  Expr=-(u[1]/2)+u[2]*(sqrt(3)/2)
  Fcn2 : Fcn  Expr=-(u[1]/2)-u[2]*(sqrt(3)/2)
  Mux : Mux  Inputs=3
  Vabcr : Outport
  wires:
  Mux/1 -> Vabcr/1
  V Dr/Qr/1 -> Fcn2/1, Fcn1/1, Fcn/1
  Fcn/1 -> Mux/1
  Fcn1/1 -> Mux/2
  Fcn2/1 -> Mux/3

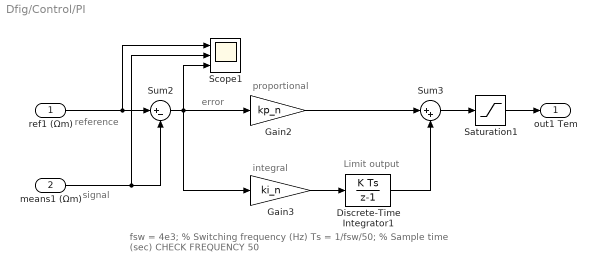
== system Dfig/Control/PI ==
  note: Limit output
  note: proportional
  note: reference
  note: error
  note: fsw = 4e3;                  % Switching frequency (Hz)
      | Ts = 1/fsw/50;            % Sample time (sec) CHECK FREQUENCY 50
  note: signal
  note: integral
  "ref1 (Ωm) " : Inport
  "means1 (Ωm) " : Inport  Port=2
  Discrete-Time Integrator1 : DiscreteIntegrator  SampleTime=1/fsw  LimitOutput=on  UpperSaturationLimit=Tem  LowerSaturationLimit=-Tem  ICPrevOutput=DiscIntNeverNeededParam  ICPrevScaledInput=DiscIntNeverNeededParam
  Gain2 : Gain  Gain=kp_n
  Gain3 : Gain  Gain=ki_n
  Saturation1 : Saturate  UpperLimit=Tem  LowerLimit=-Tem
  Scope1 : Scope  NumInputPorts=3
      settings: TimeRange=auto  MaxDataPoints=5000  SaveToWorkspace=off  SaveName=ScopeData2  YMin=-21.59845~-5~-5  YMax=194.38605~5~5  SampleInput=on  SampleTime=1/fsw
  Sum2 : Sum  Inputs=|+-
  Sum3 : Sum  Inputs=|++
  out1 Tem : Outport
  wires:
  Gain2/1 -> Sum3/1
  Sum3/1 -> Saturation1/1
  "ref1 (Ωm) "/1 -> Scope1/1, Sum2/1
  "means1 (Ωm) "/1 -> Scope1/2, Sum2/2
  Sum2/1 -> Scope1/3, Gain3/1, Gain2/1
  Gain3/1 -> Discrete-Time Integrator1/1
  Discrete-Time Integrator1/1 -> Sum3/2
  Saturation1/1 -> out1 Tem/1

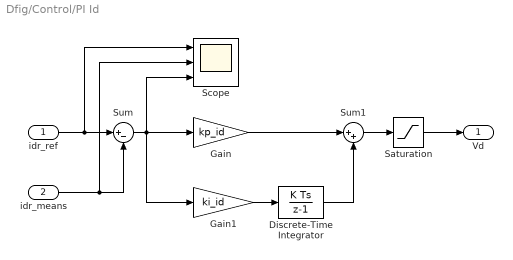
== system Dfig/Control/PI Id ==
  idr_ref : Inport
  idr_means : Inport  Port=2
  Discrete-Time Integrator : DiscreteIntegrator  SampleTime=1/fsw  LimitOutput=on  UpperSaturationLimit=Vbus/sqrt(3)  LowerSaturationLimit=-Vbus/sqrt(3)  ICPrevOutput=DiscIntNeverNeededParam  ICPrevScaledInput=DiscIntNeverNeededParam
  Gain : Gain  Gain=kp_id
  Gain1 : Gain  Gain=ki_id
  Saturation : Saturate  UpperLimit=Vbus/sqrt(3)  LowerLimit=-Vbus/sqrt(3)
  Scope : Scope  NumInputPorts=3
      settings: TimeRange=auto  MaxDataPoints=5000  SaveToWorkspace=off  YMin=-14704.68799~-5~-5  YMax=14704.68799~5~5  SampleTime=-1
  Sum : Sum  Inputs=|+-
  Sum1 : Sum  Inputs=|++
  Vd : Outport
  wires:
  idr_means/1 -> Scope/2, Sum/2
  idr_ref/1 -> Scope/1, Sum/1
  Sum/1 -> Scope/3, Gain1/1, Gain/1
  Gain/1 -> Sum1/1
  Gain1/1 -> Discrete-Time Integrator/1
  Discrete-Time Integrator/1 -> Sum1/2
  Sum1/1 -> Saturation/1
  Saturation/1 -> Vd/1

== system Dfig/Control/PI Iq ==
  iqr_ref : Inport
  iqr_means : Inport  Port=2
  Discrete-Time Integrator : DiscreteIntegrator  SampleTime=1/fsw  LimitOutput=on  UpperSaturationLimit=Vbus/sqrt(3)  LowerSaturationLimit=-Vbus/sqrt(3)  ICPrevOutput=DiscIntNeverNeededParam  ICPrevScaledInput=DiscIntNeverNeededParam
  Gain : Gain  Gain=kp_iq
  Gain1 : Gain  Gain=ki_iq
  Saturation : Saturate  UpperLimit=Vbus/sqrt(3)  LowerLimit=-Vbus/sqrt(3)
  Sum : Sum  Inputs=|+-
  Sum1 : Sum  Inputs=|++
  Vq : Outport
  wires:
  iqr_means/1 -> Sum/2
  iqr_ref/1 -> Sum/1
  Sum/1 -> Gain1/1, Gain/1
  Gain/1 -> Sum1/1
  Gain1/1 -> Discrete-Time Integrator/1
  Discrete-Time Integrator/1 -> Sum1/2
  Sum1/1 -> Saturation/1
  Saturation/1 -> Vq/1

== system Dfig/Control/abc -> DQ  ==
  note: iQr
  note: iDr
  iabcr : Inport
  Fcn : Fcn  Expr=2/3*(u[1]-u[2]/2-u[3]/2)
  Fcn1 : Fcn  Expr=2/3*(u[2]*(sqrt(3)/2)-u[3]*(sqrt(3)/2))
  Mux : Mux  Inputs=2
  i Dr/Qr : Outport
  wires:
  Mux/1 -> i Dr/Qr/1
  iabcr/1 -> Fcn1/1, Fcn/1
  Fcn/1 -> Mux/1
  Fcn1/1 -> Mux/2

== system Dfig/Control/d//q -> D//Q  ==
  Vdr_ref  Vqr_ref : Inport
  theta_r (θr) : Inport  Port=2
  Fcn : Fcn  Expr=u(1)*cos(u[3])-u[2]*sin(u[3])
  Fcn1 : Fcn  Expr=u(1)*sin(u[3])+u[2]*cos(u[3])
  Mux : Mux  Inputs=2
  Mux1 : Mux  Inputs=2
  V Dr/Qr : Outport
  wires:
  Mux/1 -> V Dr/Qr/1
  Fcn/1 -> Mux/1
  Fcn1/1 -> Mux/2
  Vdr_ref  Vqr_ref/1 -> Mux1/1
  theta_r (θr)/1 -> Mux1/2
  Mux1/1 -> Fcn/1, Fcn1/1

== system Dfig/Control1/ Angle Rotor ==
  note: V αβ
  Grid_Voltage (Vabcg) : Inport
  "Clarke: abc -> αβ " : Subsystem
  Demux : Demux  Outputs=2
  θv=tan^(-1) (Vβ/Vα) : Trigonometry  Operator=atan2
  theta_g (θg) : Outport
  tag scope: Vgalfa_beta=global
  wires:
  "Clarke: abc -> αβ "/1("Valfa/beta ") -> [Vgalfa_beta], Demux/1
  Demux/1 -> θv=tan^(-1) (Vβ/Vα)/2
  Demux/2 -> θv=tan^(-1) (Vβ/Vα)/1
  Grid_Voltage (Vabcg)/1 -> "Clarke: abc -> αβ "/1(Vabc)
  θv=tan^(-1) (Vβ/Vα)/1 -> theta_g (θg)/1

== system Dfig/Control1/3er Harmonic Inyection ==
  in : Inport
  Gain : Gain  Gain=-0.5
  MinMax : MinMax
  MinMax1 : MinMax  Function=max
  Scope : Scope
      settings: TimeRange=auto  MaxDataPoints=5000  SaveToWorkspace=off  SaveName=ScopeData2  YMin=-208.5095  YMax=235.47421  SampleTime=-1
  Sum : Sum  Inputs=|++
  Sum1 : Sum  Inputs=|++
  out : Outport
  wires:
  Gain/1 -> Sum1/2, Scope/1
  Sum/1 -> Gain/1
  Sum1/1 -> out/1
  MinMax1/1 -> Sum/2
  MinMax/1 -> Sum/1
  in/1 -> MinMax/1, MinMax1/1, Sum1/1

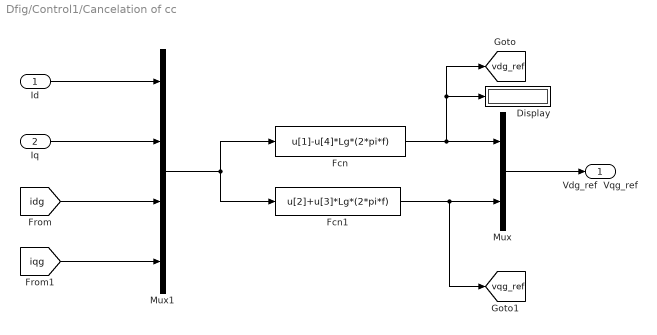
== system Dfig/Control1/Cancelation of cc ==
  Id : Inport
  Iq : Inport  Port=2
  Display : Display
  Fcn : Fcn  Expr=u[1]-u[4]*Lg*(2*pi*f)
  Fcn1 : Fcn  Expr=u[2]+u[3]*Lg*(2*pi*f)
  Mux : Mux  Inputs=2
  Mux1 : Mux
  Vdg_ref  Vqg_ref : Outport
  tag scope: vdg_ref=global, vqg_ref=global
  wires:
  [iqg] -> Mux1/4
  [idg] -> Mux1/3
  Mux1/1 -> Fcn/1, Fcn1/1
  Iq/1 -> Mux1/2
  Id/1 -> Mux1/1
  Fcn1/1 -> Mux/2, [vqg_ref]
  Fcn/1 -> Mux/1, Display/1, [vdg_ref]
  Mux/1 -> Vdg_ref  Vqg_ref/1

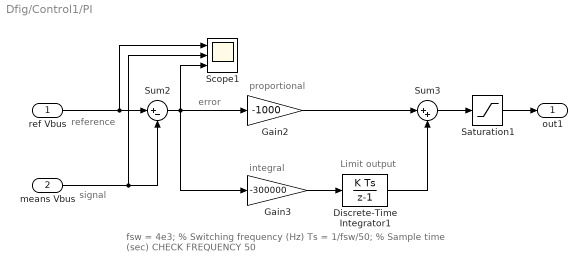
== system Dfig/Control1/PI ==
  note: integral
  note: signal
  note: fsw = 4e3;                  % Switching frequency (Hz)
      | Ts = 1/fsw/50;            % Sample time (sec) CHECK FREQUENCY 50
  note: error
  note: reference
  note: proportional
  note: Limit output
  "ref Vbus " : Inport
  "means Vbus " : Inport  Port=2
  Discrete-Time Integrator1 : DiscreteIntegrator  SampleTime=1/fsw  LimitOutput=on  UpperSaturationLimit=Ps  LowerSaturationLimit=-Ps  ICPrevOutput=DiscIntNeverNeededParam  ICPrevScaledInput=DiscIntNeverNeededParam
  Gain2 : Gain  Gain=-1000
  Gain3 : Gain  Gain=-300000
  Saturation1 : Saturate  UpperLimit=Ps  LowerLimit=-Ps
  Scope1 : Scope  NumInputPorts=3
      settings: TimeRange=auto  MaxDataPoints=5000  SaveToWorkspace=off  SaveName=ScopeData2  YMin=-2389.15954~-5~-5  YMax=3389.15954~5~5  SampleInput=on  SampleTime=1/fsw
  Sum2 : Sum  Inputs=|+-
  Sum3 : Sum  Inputs=|++
  out1 : Outport
  wires:
  Saturation1/1 -> out1/1
  Discrete-Time Integrator1/1 -> Sum3/2
  Gain3/1 -> Discrete-Time Integrator1/1
  Sum2/1 -> Gain2/1, Gain3/1, Scope1/3
  "means Vbus "/1 -> Sum2/2, Scope1/2
  "ref Vbus "/1 -> Sum2/1, Scope1/1
  Sum3/1 -> Saturation1/1
  Gain2/1 -> Sum3/1

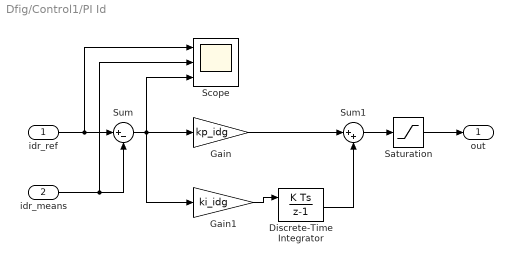
== system Dfig/Control1/PI Id ==
  idr_ref : Inport
  idr_means : Inport  Port=2
  Discrete-Time Integrator : DiscreteIntegrator  InitialConditionSource=external  SampleTime=1/fsw  LimitOutput=on  UpperSaturationLimit=Vbus/sqrt(3)  LowerSaturationLimit=-Vbus/sqrt(3)  ICPrevOutput=DiscIntNeverNeededParam  ICPrevScaledInput=DiscIntNeverNeededParam
  Gain : Gain  Gain=kp_idg
  Gain1 : Gain  Gain=ki_idg
  Saturation : Saturate  UpperLimit=Vbus/sqrt(3)*2  LowerLimit=-Vbus/sqrt(3)*2
  Scope : Scope  NumInputPorts=3
      settings: TimeRange=auto  MaxDataPoints=5000  SaveToWorkspace=off  YMin=-2140.43801~-5~-5  YMax=3453.63797~5~5  SampleTime=-1
  Sum : Sum  Inputs=|+-
  Sum1 : Sum  Inputs=|++
  out : Outport
  wires:
  Saturation/1 -> out/1
  Sum1/1 -> Saturation/1
  Discrete-Time Integrator/1 -> Sum1/2
  Gain1/1 -> Discrete-Time Integrator/1
  Gain/1 -> Sum1/1
  Sum/1 -> Gain/1, Gain1/1, Scope/3
  idr_ref/1 -> Sum/1, Scope/1
  idr_means/1 -> Sum/2, Scope/2

== system Dfig/Control1/PI Iq ==
  iqr_ref : Inport
  iqr_means : Inport  Port=2
  Discrete-Time Integrator : DiscreteIntegrator  SampleTime=1/fsw  LimitOutput=on  UpperSaturationLimit=Vbus/sqrt(3)  LowerSaturationLimit=-Vbus/sqrt(3)  ICPrevOutput=DiscIntNeverNeededParam  ICPrevScaledInput=DiscIntNeverNeededParam
  Gain : Gain  Gain=kp_iqg
  Gain1 : Gain  Gain=ki_iqg
  Saturation : Saturate  UpperLimit=Vbus/sqrt(3)  LowerLimit=-Vbus/sqrt(3)
  Sum : Sum  Inputs=|+-
  Sum1 : Sum  Inputs=|++
  out : Outport
  wires:
  Saturation/1 -> out/1
  Sum1/1 -> Saturation/1
  Discrete-Time Integrator/1 -> Sum1/2
  Gain1/1 -> Discrete-Time Integrator/1
  Gain/1 -> Sum1/1
  Sum/1 -> Gain/1, Gain1/1
  iqr_ref/1 -> Sum/1
  iqr_means/1 -> Sum/2

== system Dfig/Control1/abc -> α//β  ==
  note: iαg
  note: iβg
  iabcg : Inport
  Fcn : Fcn  Expr=2/3*(u[1]-u[2]/2-u[3]/2)
  Fcn1 : Fcn  Expr=2/3*(u[2]*(sqrt(3)/2)-u[3]*(sqrt(3)/2))
  Mux : Mux  Inputs=2
  iαg/iβg : Outport
  wires:
  Fcn1/1 -> Mux/2
  Fcn/1 -> Mux/1
  iabcg/1 -> Fcn/1, Fcn1/1
  Mux/1 -> iαg/iβg/1

== system Dfig/Control1/d//q -> α//β  ==
  Vdg_ref  Vqg_ref : Inport
  theta_g (θg) : Inport  Port=2
  Fcn : Fcn  Expr=u(1)*cos(u[3])-u[2]*sin(u[3])
  Fcn1 : Fcn  Expr=u(1)*sin(u[3])+u[2]*cos(u[3])
  Mux : Mux  Inputs=2
  Mux1 : Mux  Inputs=2
  V α/β : Outport
  wires:
  Mux1/1 -> Fcn1/1, Fcn/1
  theta_g (θg)/1 -> Mux1/2
  Vdg_ref  Vqg_ref/1 -> Mux1/1
  Fcn1/1 -> Mux/2
  Fcn/1 -> Mux/1
  Mux/1 -> V α/β/1

== system Dfig/Control1/α//β -> abc ==
  V α/β : Inport
  Fcn : Fcn  Expr=u(1)
  Fcn1 : Fcn  Expr=-(u[1]/2)+u[2]*(sqrt(3)/2)
  Fcn2 : Fcn  Expr=-(u[1]/2)-u[2]*(sqrt(3)/2)
  Mux : Mux  Inputs=3
  Vabcg : Outport
  wires:
  Fcn2/1 -> Mux/3
  Fcn1/1 -> Mux/2
  Fcn/1 -> Mux/1
  V α/β/1 -> Fcn/1, Fcn1/1, Fcn2/1
  Mux/1 -> Vabcg/1

== system Dfig/Control1/α//β -> d//q ==
  iαg/iβg : Inport
  theta_g (θg) : Inport  Port=2
  Fcn : Fcn  Expr=u(1)*cos(u[3])+u[2]*sin(u[3])
  Fcn1 : Fcn  Expr=-u(1)*sin(u[3])+u[2]*cos(u[3])
  Mux : Mux  Inputs=2
  Mux1 : Mux  Inputs=2
  i dg/qg : Outport
  wires:
  Mux1/1 -> Fcn/1, Fcn1/1
  theta_g (θg)/1 -> Mux1/2
  iαg/iβg/1 -> Mux1/1
  Fcn1/1 -> Mux/2
  Fcn/1 -> Mux/1
  Mux/1 -> i dg/qg/1

== system Dfig/Control/ Angle Rotor/Clarke: abc -> αβ  ==
  Vabc : Inport
  Fcn : Fcn  Expr=2/3*(u[1]-u[2]/2-u[3]/2)
  Fcn1 : Fcn  Expr=2/3*(u[2]*(sqrt(3)/2)-u[3]*(sqrt(3)/2))
  Mux : Mux  Inputs=2
  "Valfa/beta " : Outport
  wires:
  Mux/1 -> "Valfa/beta "/1
  Vabc/1 -> Fcn1/1, Fcn/1
  Fcn/1 -> Mux/1
  Fcn1/1 -> Mux/2

== system Dfig/Control1/ Angle Rotor/Clarke: abc -> αβ  ==
  Vabc : Inport
  Fcn : Fcn  Expr=2/3*(u[1]-u[2]/2-u[3]/2)
  Fcn1 : Fcn  Expr=2/3*(u[2]*(sqrt(3)/2)-u[3]*(sqrt(3)/2))
  Mux : Mux  Inputs=2
  "Valfa/beta " : Outport
  wires:
  Fcn1/1 -> Mux/2
  Fcn/1 -> Mux/1
  Vabc/1 -> Fcn/1, Fcn1/1
  Mux/1 -> "Valfa/beta "/1
